simulink model "model5"  (R2022a)
settings: Solver=VariableStepAuto  StartTime=0.0  StopTime=15  RelTol=1e-3
values from neighbouring files (symbols this model uses):
  A_d = sys_d.A    [config4.m]    (also in config5.m)
  B_d = sys_d.B    [config4.m]    (also in config5.m)
  Gamma_f = 1    [config5.m]
  Gamma_g = [0 1 ... (first row only)    [config5.m]
  H_f = 1    [config5.m]
  K_oc = -H_d/M    [config5.m]
  L = (H_z/M_z)'    [task4.m]    (also in task5.m)
  T = 0.2    [config4.m]    (also in config5.m)
  xi_f0 = f_0    (= 5.3)    [config5.m]
  xi_g0 = [0 ... (first row only)    [config5.m]
undefined symbols (not defined in the file or in its folder): A, B, C, L_f, L_g
settings Model: Creator=Vvlad  LastModifiedBy=Vvlad

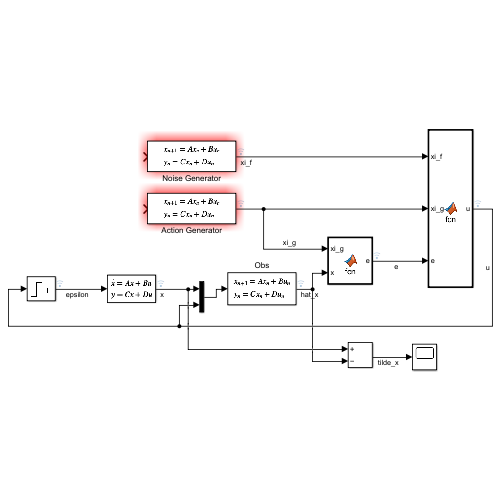
[thumbnail: Simulink's stored preview of the top-level diagram]
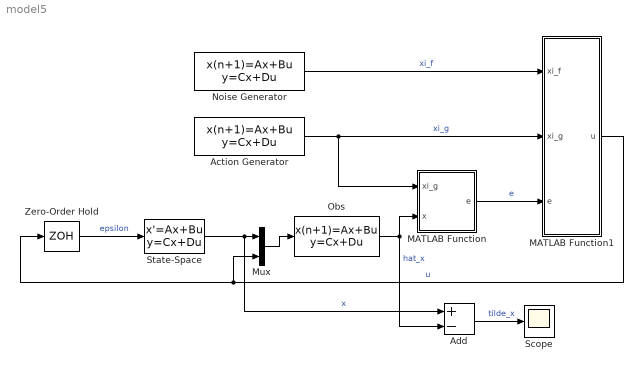
== system model5 ==
  Action Generator : DiscreteStateSpace  A=Gamma_g  B=[0;0]  C=eye(2)  D=[0;0]  InitialCondition=xi_g0  SampleTime=T
  Add : Sum  Inputs=+-
  MATLAB Function : MATLAB Function  TreatAsAtomicUnit=on
  MATLAB Function1 : MATLAB Function  TreatAsAtomicUnit=on
  Mux : Mux  Inputs=2
  Noise Generator : DiscreteStateSpace  A=Gamma_f  B=0  C=H_f  D=0  InitialCondition=xi_f0  SampleTime=T
  Obs : DiscreteStateSpace  A=A_d - L*C  B=[L*C B_d]  C=eye(2)  D=zeros(2, 3)  SampleTime=T
  Scope : Scope
  State-Space : StateSpace  A=A  B=B  C=eye(2)  D=[0;0]  InitialCondition=0
  Zero-Order Hold : ZeroOrderHold  SampleTime=-1
  wires:
  Noise Generator/1 -> MATLAB Function1/1(xi_f)  "xi_f"
  Zero-Order Hold/1 -> State-Space/1  "epsilon"
  MATLAB Function1/1(u) -> Mux/2, Zero-Order Hold/1  "u"
  Action Generator/1 -> MATLAB Function1/2(xi_g), MATLAB Function/1(xi_g)  "xi_g"
  MATLAB Function/1(e) -> MATLAB Function1/3(e)  "e"
  State-Space/1 -> Add/1, Mux/1  "x"
  Mux/1 -> Obs/1
  Obs/1 -> Add/2, MATLAB Function/2(x)  "hat_x"
  Add/1 -> Scope/1  "tilde_x"

== matlab function model5/MATLAB Function1 ==
  data: xi_f input; u output; xi_g input; e input; L_f parameter; L_g parameter; K_oc parameter
function u = fcn(xi_f, xi_g, e, L_f, L_g, K_oc)

u =  K_oc*e + L_g*xi_g - L_f*xi_f;

== matlab function model5/MATLAB Function ==
  data: xi_g input; e output; x input; M_g parameter
function e = fcn(xi_g, x, M_g)

e = M_g*xi_g - x;
